simulink model "Wiper_System"  (R2023a)
settings: Solver=FixedStepDiscrete  StartTime=0.0  StopTime=20  FixedStep=0.01  RelTol=1e-3
model workspace (MAT data in the model file):
  High_Speed_PWM_Index = 7
  Low_Speed_PWM_Index = 0
  PWM = [0 0.4 0.45 0.5 0.55 0.6 0.65 0.7]
libraries: simulink x1, SignalEditorBlockLib x1
settings Model: Creator=AIO  LastModifiedBy=AIO
settings OptimizationCC: DefaultParameterBehavior=Inlined  EnhancedBackFolding=on  PassReuseOutputArgsAs=Individual arguments  ZeroExternalMemoryAtStartup=off  ZeroInternalMemoryAtStartup=off  OptimizeBlockOrder=speed  DifferentSizesBufferReuse=on  OptimizationCustomize=off  EfficientTunableParamExpr=on
settings DebuggingCC: ParameterTunabilityLossMsg=error
settings SFSimCC: MATLABDynamicMemAlloc=off
settings RTWCC: Description=Embedded Coder  SystemTargetFile=ert.tlc  TemplateMakefile=ert_default_tmf
settings CodeAppCC: ForceParamTrailComments=on  IgnoreCustomStorageClasses=off  OperatorAnnotations=on  SimulinkDataObjDesc=on  SFDataObjDesc=on  InsertBlockDesc=on
settings ERTTargetCC: TargetLangStandard=C99 (ISO)  GenerateSampleERTMain=on  SupportContinuousTime=on  InlinedParameterPlacement=NonHierarchical  ERTCustomFileTemplate=example_file_process.tlc

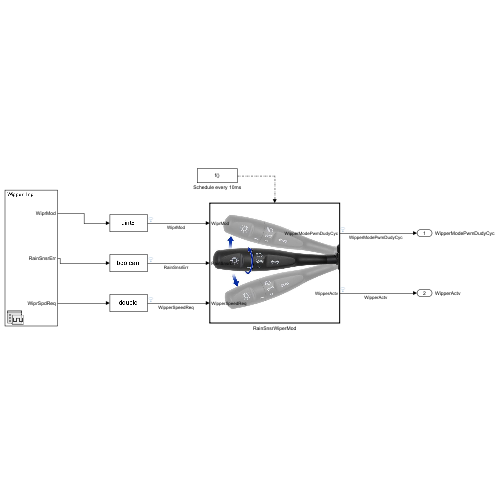
[thumbnail: Simulink's stored preview of the top-level diagram]
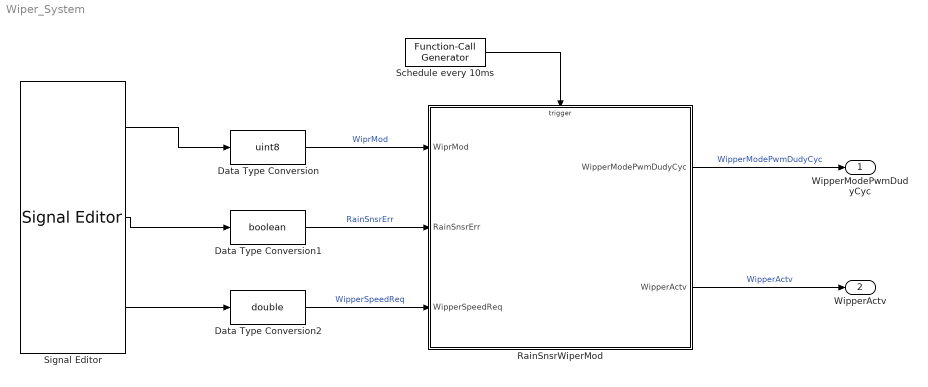
== system Wiper_System ==
  Data Type Conversion : DataTypeConversion  OutDataTypeStr=uint8  SaturateOnIntegerOverflow=off  RndMeth=Floor
  Data Type Conversion1 : DataTypeConversion  OutDataTypeStr=boolean  SaturateOnIntegerOverflow=off  RndMeth=Floor
  Data Type Conversion2 : DataTypeConversion  OutDataTypeStr=double  SaturateOnIntegerOverflow=off  RndMeth=Floor
  RainSnsrWiperMod : Subsystem
      mask Display: image('C:\Users\AIO\Downloads\WhatsApp Image 2024-01-20 at 8.16.46 PM.jpeg'); % Use "Edit Image" on toolstrip to change.
  Schedule every 10ms : simulink/Ports & Subsystems/Function-Call Generator  sample_time=10e-3  numberOfIterations=1  DisallowWideOutput=off
  Signal Editor : SignalEditorBlockLib/Signal Editor  FileName=Signal_Input_Test.mat  ActiveScenario=Wipper_Inp  ActiveSignal=WiprMod  IsBus=off  OutputBusObjectStr=Bus: BusObject  SampleTime=0  Interpolate=off  ZeroCross=off  OutputAfterFinalValue=Setting to zero  Unit=inherit  PreserveSignalName=on  ApplySigPropsToAllScenarios=on
  WipperModePwmDudyCyc : Outport
  WipperActv : Outport  Port=2
  wires:
  Schedule every 10ms/1 -> RainSnsrWiperMod/Trigger
  RainSnsrWiperMod/1(WipperModePwmDudyCyc) -> WipperModePwmDudyCyc/1  "WipperModePwmDudyCyc"
  RainSnsrWiperMod/2(WipperActv) -> WipperActv/1  "WipperActv"
  Signal Editor/1 -> Data Type Conversion/1
  Signal Editor/2 -> Data Type Conversion1/1
  Data Type Conversion/1 -> RainSnsrWiperMod/1(WiprMod)  "WiprMod"
  Data Type Conversion1/1 -> RainSnsrWiperMod/2(RainSnsrErr)  "RainSnsrErr"
  Signal Editor/3 -> Data Type Conversion2/1
  Data Type Conversion2/1 -> RainSnsrWiperMod/3(WipperSpeedReq)  "WipperSpeedReq"

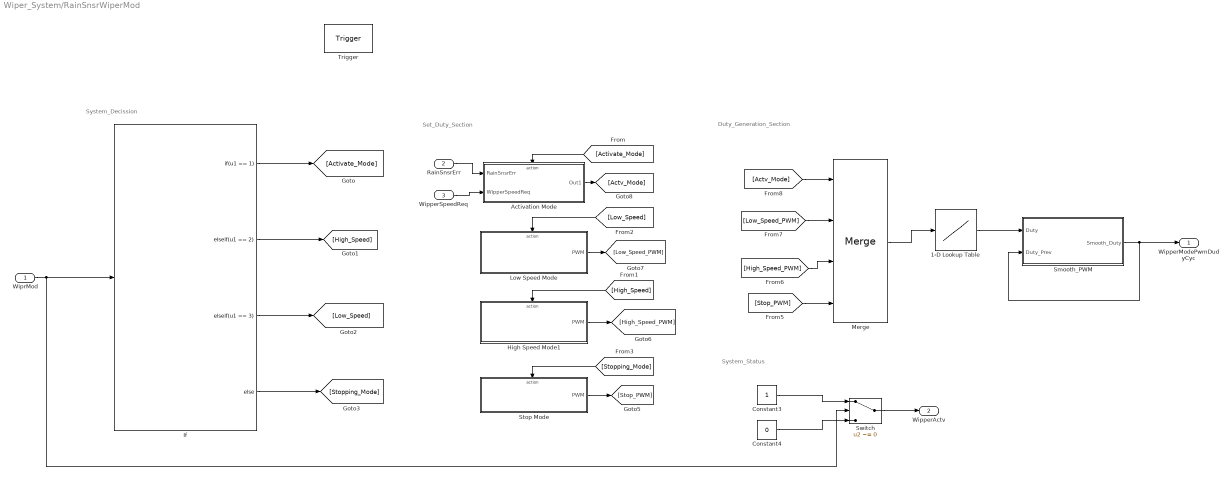
== system Wiper_System/RainSnsrWiperMod ==
  note: System_Status
  note: Duty_Generation_Section
  note: Set_Duty_Section
  note: System_Decission
  WiprMod : Inport
  RainSnsrErr : Inport  Port=2  OutDataTypeStr=boolean
  WipperSpeedReq : Inport  Port=3
  Trigger : TriggerPort  TriggerType=function-call  VariantControl=(inherit)  PortDimensions=1
  1-D Lookup Table : Lookup_n-D  NumberOfTableDimensions=1  BreakpointsForDimension1=[0:7]  Table=PWM  InternalRulePriority=Speed  RndMeth=Simplest
  Activation Mode : Subsystem  TreatAsAtomicUnit=on
  Constant3 : Constant
  Constant4 : Constant  Value=0
  High Speed Mode1 : Subsystem  TreatAsAtomicUnit=on
  If : If  IfExpression=u1 == 1  ElseIfExpressions=u1 == 2,u1 == 3
  Low Speed Mode : Subsystem  TreatAsAtomicUnit=on
  Merge : Merge  Inputs=4
  Smooth_PWM : Subsystem
  Stop Mode : Subsystem  TreatAsAtomicUnit=on
  Switch : Switch  Criteria=u2 ~= 0  SaturateOnIntegerOverflow=off  InputSameDT=off
  WipperModePwmDudyCyc : Outport
  WipperActv : Outport  Port=2
  wires:
  WiprMod/1 -> Switch/2, If/1
  Constant3/1 -> Switch/1
  Constant4/1 -> Switch/3
  Switch/1 -> WipperActv/1
  If/1 -> [Activate_Mode]
  If/3 -> [Low_Speed]
  If/4 -> [Stopping_Mode]
  If/2 -> [High_Speed]
  [Stop_PWM] -> Merge/4
  [High_Speed_PWM] -> Merge/3
  [Low_Speed_PWM] -> Merge/2
  [Actv_Mode] -> Merge/1
  [Activate_Mode] -> Activation Mode/Action
  [Low_Speed] -> Low Speed Mode/Action
  Activation Mode/1(Out1) -> [Actv_Mode]
  [High_Speed] -> High Speed Mode1/Action
  [Stopping_Mode] -> Stop Mode/Action
  Low Speed Mode/1(PWM) -> [Low_Speed_PWM]
  High Speed Mode1/1(PWM) -> [High_Speed_PWM]
  Stop Mode/1(PWM) -> [Stop_PWM]
  Merge/1 -> 1-D Lookup Table/1
  RainSnsrErr/1 -> Activation Mode/1(RainSnsrErr)
  WipperSpeedReq/1 -> Activation Mode/2(WipperSpeedReq)
  1-D Lookup Table/1 -> Smooth_PWM/1(Duty)
  Smooth_PWM/1(Smooth_Duty) -> Smooth_PWM/2(Duty_Prev), WipperModePwmDudyCyc/1

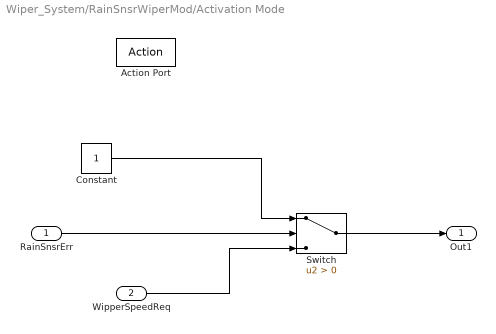
== system Wiper_System/RainSnsrWiperMod/Activation Mode ==
  RainSnsrErr : Inport
  WipperSpeedReq : Inport  Port=2
  Action Port : ActionPort  ActionPortLabel=if(u1 == 1)
  Constant : Constant
  Switch : Switch  Criteria=u2 > Threshold  SaturateOnIntegerOverflow=off  InputSameDT=off
  Out1 : Outport
  wires:
  RainSnsrErr/1 -> Switch/2
  Constant/1 -> Switch/1
  Switch/1 -> Out1/1
  WipperSpeedReq/1 -> Switch/3

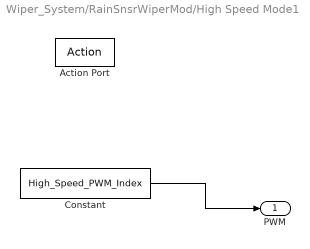
== system Wiper_System/RainSnsrWiperMod/High Speed Mode1 ==
  Action Port : ActionPort  ActionPortLabel=elseif(u1 == 2)
  Constant : Constant  Value=High_Speed_PWM_Index
  PWM : Outport
  wires:
  Constant/1 -> PWM/1

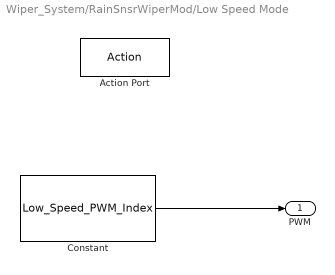
== system Wiper_System/RainSnsrWiperMod/Low Speed Mode ==
  Action Port : ActionPort  ActionPortLabel=elseif(u1 == 3)
  Constant : Constant  Value=Low_Speed_PWM_Index
  PWM : Outport
  wires:
  Constant/1 -> PWM/1

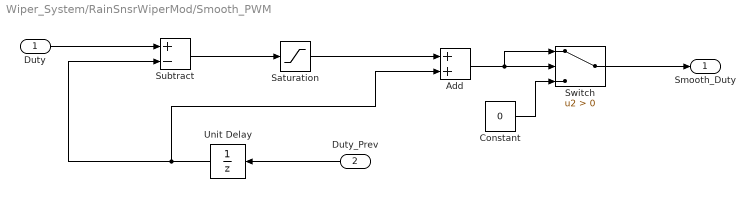
== system Wiper_System/RainSnsrWiperMod/Smooth_PWM ==
  Duty : Inport
  Duty_Prev : Inport  Port=2
  Add : Sum
  Constant : Constant  Value=0
  Saturation : Saturate  UpperLimit=0.005  LowerLimit=-0.005
  Subtract : Sum  Inputs=+-
  Switch : Switch  Criteria=u2 > Threshold  SaturateOnIntegerOverflow=off  InputSameDT=off
  Unit Delay : UnitDelay  SampleTime=-1  HasFrameUpgradeWarning=on
  Smooth_Duty : Outport
  wires:
  Duty/1 -> Subtract/1
  Subtract/1 -> Saturation/1
  Saturation/1 -> Add/1
  Duty_Prev/1 -> Unit Delay/1
  Unit Delay/1 -> Add/2, Subtract/2
  Add/1 -> Switch/1, Switch/2
  Switch/1 -> Smooth_Duty/1
  Constant/1 -> Switch/3

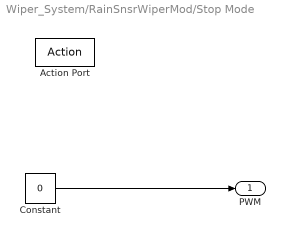
== system Wiper_System/RainSnsrWiperMod/Stop Mode ==
  Action Port : ActionPort  ActionPortLabel=else
  Constant : Constant  Value=0
  PWM : Outport
  wires:
  Constant/1 -> PWM/1
